simulink model "model_QK_SFSVD_ROS"  (Simulink 7.6)
settings: Solver=FixedStepDiscrete  SolverMode=SingleTasking  StartTime=0  StopTime=100  FixedStep=0.01  RelTol=1e-3
values from neighbouring files (symbols this model uses):
  parameter = block.DialogPrm(3).Data    [Kalmangain.m]    (also in init_QK_ROS.m = load('parameter'); statePrediction.m = block.DialogPrm(2).Data)
libraries: PortLib x11, simulink x2, aerolibutil x2
(part 4 of 4)

== matlab function Kalmanfilter/correction ==
  data: xpred input double; x output double; Ppred input double; y input double; sensors input double; P output double; parameter parameter double
function [x,P] = correction(xpred, Ppred, y, sensors, parameter)


R0   = parameter.R0;
Pos0 = parameter.Pos0;
B0   = parameter.B0;

x    = xpred;
P    = Ppred;
% Horizontal GPS Position
if sensors(1) == 1
    [temp, C, R] = getGPSPosition(xpred,y(1:2),R0(1:2),Pos0);
    K            = Ppred*C'*(C*Ppred*C'  +  R)^( - 1);
    x            = x  +  K*temp;
    P            = (eye(length(xpred))  -  K*C)*P;
end
% Barometric height
if sensors(2) == 1
    [temp,C,R]  =  getBarometer(xpred,y(3),R0(3));
    K           = Ppred*C'*(C*Ppred*C'  +  R)^( - 1);
    x           = x  +  K*temp;
    P           = (eye(length(xpred))  -  K*C)*P;
end
% GPS Velocity
if sensors(3) == 1
    [temp,C,R]  =  getGPSVelocity(xpred,y(4:6),R0(4:6));
    K           = Ppred*C'*(C*Ppred*C'  +  R)^( - 1);
    x           = x  +  K*temp;
    P           = (eye(length(xpred))  -  K*C)*P;
end
% Acceleration
if sensors(4) == 1
    [temp,C,R]  =  getAccelerometer(xpred,y(7:9),R0(7:9),parameter);
    K           = Ppred*C'*(C*Ppred*C'  +  R)^( - 1);
    x           = x  +  K*temp;
    P           = (eye(length(xpred))  -  K*C)*P;
end
% Gyroscope
if sensors(5) == 1
    [temp,C,R]  =  getGyroscope(xpred,y(10:12),R0(10:12));
    K           = Ppred*C'*(C*Ppred*C'  +  R)^( - 1);
    x           = x  +  K*temp;
    P           = (eye(length(xpred))  -  K*C)*P;
end
% Omega motor
if sensors(6) == 1
    [temp,C,R]  =  getOmegaMotor(xpred,y(13:16),R0(13:16));
    K           = Ppred*C'*(C*Ppred*C'  +  R)^( - 1);
    x           = x  +  K*temp;
    P           = (eye(length(xpred))  -  K*C)*P;
end
% Magnetometer
if sensors(7) == 1
    [temp, C, R] = getMagneticField(xpred,y(17:19),R0(17:19),B0);
    K            = Ppred*C'*(C*Ppred*C'  +  R)^( - 1);
    x            = x  +  K*temp;
    P            = (eye(length(xpred))  -  K*C)*P;
end
% normalize quaternions
q_0 = x(7);
q_1 = x(8);
q_2 = x(9);
q_3 = x(10);
q_length = sqrt((q_0*q_0) + (q_1*q_1) + (q_2*q_2) + (q_3*q_3));

x(7)  = x(7)/q_length;
x(8)  = x(8)/q_length;
x(9)  = x(9)/q_length;
x(10) = x(10)/q_length;

%endfunction

function [temp, C, R] = getGPSPosition(x,real_measurements,Rin,Pos0)

y = zeros(2,1);
C = zeros(2,31);
R = zeros(2);

y(1)   = Pos0(1)  +  x(1)/6378137.0/pi*180.0;                         % Latitude
y(2)   = Pos0(2)  +  x(2)/6378137.0/pi/cos(Pos0(1)*pi/180.0)*180.0;   % Longitude

C(1,1) = 180/6378137/pi;
C(2,2) = 180/6378137/pi/cos(Pos0(1)*pi/180);

R(1,1) = 180*Rin(1)/6378137/pi;
R(2,2) = 180*Rin(2)/6378137/pi/cos(Pos0(1)*pi/180);

temp   = real_measurements  -  y;

function [temp, C, R] = getGPSVelocity(x,real_measurements,Rin)

y = zeros(3,1);
C = zeros(3,31);

u = x(4);
v = x(5);
w = x(6);
q_0 = x(7);
q_1 = x(8);
q_2 = x(9);
q_3 = x(10);

y(1) = u*(q_0*q_0 + q_1*q_1 - q_2*q_2 - q_3*q_3) - v*(q_0*q_3*2.0 - q_1*q_2*2.0) + w*(q_0*q_2*2.0 + q_1*q_3*2.0);
y(2) = v*(q_0*q_0 - q_1*q_1 + q_2*q_2 - q_3*q_3) + u*(q_0*q_3*2.0 + q_1*q_2*2.0) - w*(q_0*q_1*2.0 - q_2*q_3*2.0);
y(3) = w*(q_0*q_0 - q_1*q_1 - q_2*q_2 + q_3*q_3) - u*(q_0*q_2*2.0 - q_1*q_3*2.0) + v*(q_0*q_1*2.0 + q_2*q_3*2.0);

C(1,4)  = q_0*q_0 + q_1*q_1 - q_2*q_2 - q_3*q_3;
C(1,5)  = q_0*q_3* - 2.0 + q_1*q_2*2.0;
C(1,6)  = q_0*q_2*2.0 + q_1*q_3*2.0;
C(1,7)  = q_0*u*2.0 - q_3*v*2.0 + q_2*w*2.0;
C(1,8)  = q_1*u*2.0 + q_2*v*2.0 + q_3*w*2.0;
C(1,9)  = q_2*u* - 2.0 + q_1*v*2.0 + q_0*w*2.0;
C(1,10) = q_3*u* - 2.0 - q_0*v*2.0 + q_1*w*2.0;
C(2,4)  = q_0*q_3*2.0 + q_1*q_2*2.0;
C(2,5)  = q_0*q_0 - q_1*q_1 + q_2*q_2 - q_3*q_3;
C(2,6)  = q_0*q_1* - 2.0 + q_2*q_3*2.0;
C(2,7)  = q_3*u*2.0 + q_0*v*2.0 - q_1*w*2.0;
C(2,8)  = q_2*u*2.0 - q_1*v*2.0 - q_0*w*2.0;
C(2,9)  = q_1*u*2.0 + q_2*v*2.0 + q_3*w*2.0;
C(2,10) = q_0*u*2.0 - q_3*v*2.0 + q_2*w*2.0;
C(3,4)  = q_0*q_2* - 2.0 + q_1*q_3*2.0;
C(3,5)  = q_0*q_1*2.0 + q_2*q_3*2.0;
C(3,6)  = q_0*q_0 - q_1*q_1 - q_2*q_2 + q_3*q_3;
C(3,7)  = q_2*u* - 2.0 + q_1*v*2.0 + q_0*w*2.0;
C(3,8)  = q_3*u*2.0 + q_0*v*2.0 - q_1*w*2.0;
C(3,9)  = q_0*u* - 2.0 + q_3*v*2.0 - q_2*w*2.0;
C(3,10) = q_1*u*2.0 + q_2*v*2.0 + q_3*w*2.0;

R       = diag(Rin);

temp    = real_measurements  -  y;


function [temp, C, R] = getMagneticField(x,real_measurements,Rin,B)

q_0 = x(7);
q_1 = x(8);
q_2 = x(9);
q_3 = x(10);

y       = zeros(3,1);
C       = zeros(3,31);

fieldLength             = eps  +  sqrt(B(1)*B(1) + B(2)*B(2) + B(3)*B(3));
fieldLengthMeasurement  = eps  +  sqrt(real_measurements(1)^2  +  real_measurements(2)^2  +  real_measurements(3)^2);

%% Magnetometer updates only heading angle
y(1) = (B(2)*(q_0*q_3*2.0 + q_1*q_2*2.0) - B(3)*(q_0*q_2*2.0 - q_1*q_3*2.0) + B(1)*(q_0*q_0 + q_1*q_1 - q_2*q_2 - q_3*q_3))/fieldLength;
y(2) = ( - B(1)*(q_0*q_3*2.0 - q_1*q_2*2.0) + B(3)*(q_0*q_1*2.0 + q_2*q_3*2.0) + B(2)*(q_0*q_0 - q_1*q_1 + q_2*q_2 - q_3*q_3))/fieldLength;
y(3) = (B(1)*(q_0*q_2*2.0 + q_1*q_3*2.0) - B(2)*(q_0*q_1*2.0 - q_2*q_3*2.0) + B(3)*(q_0*q_0 - q_1*q_1 - q_2*q_2 + q_3*q_3))/fieldLength;

C(1,7) =  - q_3*(q_0*(B(2)*q_0*1.0/fieldLength*2.0 - B(1)*q_3*1.0/fieldLength*2.0 + B(3)*q_1*1.0/fieldLength*2.0) + q_1*(B(1)*q_2*1.0/fieldLength*2.0 - B(2)*q_1*1.0/fieldLength*2.0 + B(3)*q_0*1.0/fieldLength*2.0) + q_2*(B(1)*q_1*1.0/fieldLength*2.0 + B(2)*q_2*1.0/fieldLength*2.0 + B(3)*q_3*1.0/fieldLength*2.0) - q_3*(B(1)*q_0*1.0/fieldLength*2.0 + B(2)*q_3*1.0/fieldLength*2.0 - B(3)*q_2*1.0/fieldLength*2.0));
C(1,8) = q_2*(q_0*(B(2)*q_0*1.0/fieldLength*2.0 - B(1)*q_3*1.0/fieldLength*2.0 + B(3)*q_1*1.0/fieldLength*2.0) + q_1*(B(1)*q_2*1.0/fieldLength*2.0 - B(2)*q_1*1.0/fieldLength*2.0 + B(3)*q_0*1.0/fieldLength*2.0) + q_2*(B(1)*q_1*1.0/fieldLength*2.0 + B(2)*q_2*1.0/fieldLength*2.0 + B(3)*q_3*1.0/fieldLength*2.0) - q_3*(B(1)*q_0*1.0/fieldLength*2.0 + B(2)*q_3*1.0/fieldLength*2.0 - B(3)*q_2*1.0/fieldLength*2.0));
C(1,9) =  - q_1*(q_0*(B(2)*q_0*1.0/fieldLength*2.0 - B(1)*q_3*1.0/fieldLength*2.0 + B(3)*q_1*1.0/fieldLength*2.0) + q_1*(B(1)*q_2*1.0/fieldLength*2.0 - B(2)*q_1*1.0/fieldLength*2.0 + B(3)*q_0*1.0/fieldLength*2.0) + q_2*(B(1)*q_1*1.0/fieldLength*2.0 + B(2)*q_2*1.0/fieldLength*2.0 + B(3)*q_3*1.0/fieldLength*2.0) - q_3*(B(1)*q_0*1.0/fieldLength*2.0 + B(2)*q_3*1.0/fieldLength*2.0 - B(3)*q_2*1.0/fieldLength*2.0));
C(1,10) = q_0*(q_0*(B(2)*q_0*1.0/fieldLength*2.0 - B(1)*q_3*1.0/fieldLength*2.0 + B(3)*q_1*1.0/fieldLength*2.0) + q_1*(B(1)*q_2*1.0/fieldLength*2.0 - B(2)*q_1*1.0/fieldLength*2.0 + B(3)*q_0*1.0/fieldLength*2.0) + q_2*(B(1)*q_1*1.0/fieldLength*2.0 + B(2)*q_2*1.0/fieldLength*2.0 + B(3)*q_3*1.0/fieldLength*2.0) - q_3*(B(1)*q_0*1.0/fieldLength*2.0 + B(2)*q_3*1.0/fieldLength*2.0 - B(3)*q_2*1.0/fieldLength*2.0));
C(2,7) = q_3*(q_0*(B(1)*q_0*1.0/fieldLength*2.0 + B(2)*q_3*1.0/fieldLength*2.0 - B(3)*q_2*1.0/fieldLength*2.0) - q_2*(B(1)*q_2*1.0/fieldLength*2.0 - B(2)*q_1*1.0/fieldLength*2.0 + B(3)*q_0*1.0/fieldLength*2.0) + q_1*(B(1)*q_1*1.0/fieldLength*2.0 + B(2)*q_2*1.0/fieldLength*2.0 + B(3)*q_3*1.0/fieldLength*2.0) + q_3*(B(2)*q_0*1.0/fieldLength*2.0 - B(1)*q_3*1.0/fieldLength*2.0 + B(3)*q_1*1.0/fieldLength*2.0));
C(2,8) =  - q_2*(q_0*(B(1)*q_0*1.0/fieldLength*2.0 + B(2)*q_3*1.0/fieldLength*2.0 - B(3)*q_2*1.0/fieldLength*2.0) - q_2*(B(1)*q_2*1.0/fieldLength*2.0 - B(2)*q_1*1.0/fieldLength*2.0 + B(3)*q_0*1.0/fieldLength*2.0) + q_1*(B(1)*q_1*1.0/fieldLength*2.0 + B(2)*q_2*1.0/fieldLength*2.0 + B(3)*q_3*1.0/fieldLength*2.0) + q_3*(B(2)*q_0*1.0/fieldLength*2.0 - B(1)*q_3*1.0/fieldLength*2.0 + B(3)*q_1*1.0/fieldLength*2.0));
C(2,9) = q_1*(q_0*(B(1)*q_0*1.0/fieldLength*2.0 + B(2)*q_3*1.0/fieldLength*2.0 - B(3)*q_2*1.0/fieldLength*2.0) - q_2*(B(1)*q_2*1.0/fieldLength*2.0 - B(2)*q_1*1.0/fieldLength*2.0 + B(3)*q_0*1.0/fieldLength*2.0) + q_1*(B(1)*q_1*1.0/fieldLength*2.0 + B(2)*q_2*1.0/fieldLength*2.0 + B(3)*q_3*1.0/fieldLength*2.0) + q_3*(B(2)*q_0*1.0/fieldLength*2.0 - B(1)*q_3*1.0/fieldLength*2.0 + B(3)*q_1*1.0/fieldLength*2.0));
C(2,10) =  - q_0*(q_0*(B(1)*q_0*1.0/fieldLength*2.0 + B(2)*q_3*1.0/fieldLength*2.0 - B(3)*q_2*1.0/fieldLength*2.0) - q_2*(B(1)*q_2*1.0/fieldLength*2.0 - B(2)*q_1*1.0/fieldLength*2.0 + B(3)*q_0*1.0/fieldLength*2.0) + q_1*(B(1)*q_1*1.0/fieldLength*2.0 + B(2)*q_2*1.0/fieldLength*2.0 + B(3)*q_3*1.0/fieldLength*2.0) + q_3*(B(2)*q_0*1.0/fieldLength*2.0 - B(1)*q_3*1.0/fieldLength*2.0 + B(3)*q_1*1.0/fieldLength*2.0));
C(3,7) = q_3*( - q_0*(B(1)*q_1*1.0/fieldLength*2.0 + B(2)*q_2*1.0/fieldLength*2.0 + B(3)*q_3*1.0/fieldLength*2.0) + q_1*(B(1)*q_0*1.0/fieldLength*2.0 + B(2)*q_3*1.0/fieldLength*2.0 - B(3)*q_2*1.0/fieldLength*2.0) + q_2*(B(2)*q_0*1.0/fieldLength*2.0 - B(1)*q_3*1.0/fieldLength*2.0 + B(3)*q_1*1.0/fieldLength*2.0) + q_3*(B(1)*q_2*1.0/fieldLength*2.0 - B(2)*q_1*1.0/fieldLength*2.0 + B(3)*q_0*1.0/fieldLength*2.0));
C(3,8) =  - q_2*( - q_0*(B(1)*q_1*1.0/fieldLength*2.0 + B(2)*q_2*1.0/fieldLength*2.0 + B(3)*q_3*1.0/fieldLength*2.0) + q_1*(B(1)*q_0*1.0/fieldLength*2.0 + B(2)*q_3*1.0/fieldLength*2.0 - B(3)*q_2*1.0/fieldLength*2.0) + q_2*(B(2)*q_0*1.0/fieldLength*2.0 - B(1)*q_3*1.0/fieldLength*2.0 + B(3)*q_1*1.0/fieldLength*2.0) + q_3*(B(1)*q_2*1.0/fieldLength*2.0 - B(2)*q_1*1.0/fieldLength*2.0 + B(3)*q_0*1.0/fieldLength*2.0));
C(3,9) = q_1*( - q_0*(B(1)*q_1*1.0/fieldLength*2.0 + B(2)*q_2*1.0/fieldLength*2.0 + B(3)*q_3*1.0/fieldLength*2.0) + q_1*(B(1)*q_0*1.0/fieldLength*2.0 + B(2)*q_3*1.0/fieldLength*2.0 - B(3)*q_2*1.0/fieldLength*2.0) + q_2*(B(2)*q_0*1.0/fieldLength*2.0 - B(1)*q_3*1.0/fieldLength*2.0 + B(3)*q_1*1.0/fieldLength*2.0) + q_3*(B(1)*q_2*1.0/fieldLength*2.0 - B(2)*q_1*1.0/fieldLength*2.0 + B(3)*q_0*1.0/fieldLength*2.0));
C(3,10) =  - q_0*( - q_0*(B(1)*q_1*1.0/fieldLength*2.0 + B(2)*q_2*1.0/fieldLength*2.0 + B(3)*q_3*1.0/fieldLength*2.0) + q_1*(B(1)*q_0*1.0/fieldLength*2.0 + B(2)*q_3*1.0/fieldLength*2.0 - B(3)*q_2*1.0/fieldLength*2.0) + q_2*(B(2)*q_0*1.0/fieldLength*2.0 - B(1)*q_3*1.0/fieldLength*2.0 + B(3)*q_1*1.0/fieldLength*2.0) + q_3*(B(1)*q_2*1.0/fieldLength*2.0 - B(2)*q_1*1.0/fieldLength*2.0 + B(3)*q_0*1.0/fieldLength*2.0));

R       = diag(Rin);

temp    = real_measurements/fieldLengthMeasurement  -  y;


function [temp,C,R] = getBarometer(x,real_measurements,Rin)

%% Initial conditions
p_z = x(3);

C      = zeros(1,31);
C(1,3) = 1.0;

R       = diag(Rin);

temp    = real_measurements  -  p_z;

function [temp,C,R] = getAccelerometer(x,real_measurements,Rin,parameter)

% parameters
g     = parameter.g;
l_m   = parameter.l_m;
m     = parameter.m;
CT2s  = parameter.CT2s;
CT1s  = parameter.CT1s;
C_wz  = parameter.C_wz;

%% Initial conditions
u = x(4);
v = x(5);
w = x(6);
q_0 = x(7);
q_1 = x(8);
q_2 = x(9);
q_3 = x(10);
a_x_bias = x(11);
a_y_bias = x(12);
a_z_bias = x(13);

p = x(17);
q = x(18);
r = x(19);
w_1 = x(20);
w_2 = x(21);
w_3 = x(22);
w_4 = x(23);

CT0s = x(25);

v_x_wind = x(29);
v_y_wind = x(30);
C_wxy    = x(31);

y     = zeros(3,1);
C     = zeros(3,31);

vx_res =  - u + v_x_wind*(q_0*q_0 + q_1*q_1 - q_2*q_2 - q_3*q_3) + v_y_wind*(q_0*q_3*2.0 + q_1*q_2*2.0);
vy_res = v - v_y_wind*(q_0*q_0 - q_1*q_1 + q_2*q_2 - q_3*q_3) + v_x_wind*(q_0*q_3*2.0 - q_1*q_2*2.0);
vz_res = w - v_x_wind*(q_0*q_2*2.0 + q_1*q_3*2.0) + v_y_wind*(q_0*q_1*2.0 - q_2*q_3*2.0);
velocityLength = eps + sqrt(vx_res^2  +  vy_res^2  +  vz_res^2);


if sum(x(20:23)) < 1500 % ground contact if motor speed is to low
    y(1) = a_x_bias + g*(q_0*q_2*2.0 - q_1*q_3*2.0);
    y(2) = a_y_bias - g*(q_0*q_1*2.0 + q_2*q_3*2.0);
    y(3) = a_z_bias - g*(q_0*q_0 - q_1*q_1 - q_2*q_2 + q_3*q_3);
    
    C(1,7) = g*q_2*2.0;
    C(1,8) = g*q_3* - 2.0;
    C(1,9) = g*q_0*2.0;
    C(1,10) = g*q_1* - 2.0;
    C(1,11) = 1.0;
    C(2,7) = g*q_1* - 2.0;
    C(2,8) = g*q_0* - 2.0;
    C(2,9) = g*q_3* - 2.0;
    C(2,10) = g*q_2* - 2.0;
    C(2,12) = 1.0;
    C(3,7) = g*q_0* - 2.0;
    C(3,8) = g*q_1*2.0;
    C(3,9) = g*q_2*2.0;
    C(3,10) = g*q_3* - 2.0;
    C(3,13) = 1.0;
else
    y(1) = a_x_bias - q*w + r*v + (C_wxy*(vx_res)*velocityLength)/m;
    y(2) = a_y_bias + p*w - r*u - (C_wxy*velocityLength*(vy_res))/m;
    y(3) = a_z_bias - p*v + q*u - (CT0s*(w_1*w_1) + CT0s*(w_2*w_2) + CT0s*(w_3*w_3) + CT0s*(w_4*w_4) - CT1s*w_2*(w + l_m*p + q_0*q_1*v_y_wind*2.0 - q_0*q_2*v_x_wind*2.0 - q_1*q_3*v_x_wind*2.0 - q_2*q_3*v_y_wind*2.0) - CT1s*w_3*(w + l_m*q + q_0*q_1*v_y_wind*2.0 - q_0*q_2*v_x_wind*2.0 - q_1*q_3*v_x_wind*2.0 - q_2*q_3*v_y_wind*2.0) + CT1s*w_4*( - w + l_m*p - q_0*q_1*v_y_wind*2.0 + q_0*q_2*v_x_wind*2.0 + q_1*q_3*v_x_wind*2.0 + q_2*q_3*v_y_wind*2.0) + CT1s*w_1*( - w + l_m*q - q_0*q_1*v_y_wind*2.0 + q_0*q_2*v_x_wind*2.0 + q_1*q_3*v_x_wind*2.0 + q_2*q_3*v_y_wind*2.0) + CT2s*abs( - w + l_m*p - q_0*q_1*v_y_wind*2.0 + q_0*q_2*v_x_wind*2.0 + q_1*q_3*v_x_wind*2.0 + q_2*q_3*v_y_wind*2.0)*( - w + l_m*p - q_0*q_1*v_y_wind*2.0 + q_0*q_2*v_x_wind*2.0 + q_1*q_3*v_x_wind*2.0 + q_2*q_3*v_y_wind*2.0) + CT2s*abs( - w + l_m*q - q_0*q_1*v_y_wind*2.0 + q_0*q_2*v_x_wind*2.0 + q_1*q_3*v_x_wind*2.0 + q_2*q_3*v_y_wind*2.0)*( - w + l_m*q - q_0*q_1*v_y_wind*2.0 + q_0*q_2*v_x_wind*2.0 + q_1*q_3*v_x_wind*2.0 + q_2*q_3*v_y_wind*2.0) - CT2s*abs(w + l_m*p + q_0*q_1*v_y_wind*2.0 - q_0*q_2*v_x_wind*2.0 - q_1*q_3*v_x_wind*2.0 - q_2*q_3*v_y_wind*2.0)*(w + l_m*p + q_0*q_1*v_y_wind*2.0 - q_0*q_2*v_x_wind*2.0 - q_1*q_3*v_x_wind*2.0 - q_2*q_3*v_y_wind*2.0) - CT2s*abs(w + l_m*q + q_0*q_1*v_y_wind*2.0 - q_0*q_2*v_x_wind*2.0 - q_1*q_3*v_x_wind*2.0 - q_2*q_3*v_y_wind*2.0)*(w + l_m*q + q_0*q_1*v_y_wind*2.0 - q_0*q_2*v_x_wind*2.0 - q_1*q_3*v_x_wind*2.0 - q_2*q_3*v_y_wind*2.0))/m - (C_wz*(vz_res)*velocityLength)/m;
    
    C(1,4) =  - (C_wxy*velocityLength)/m - (C_wxy*(vx_res)*(u* - 2.0 + v_x_wind*(q_0*q_0 + q_1*q_1 - q_2*q_2 - q_3*q_3)*2.0 + v_y_wind*(q_0*q_3*2.0 + q_1*q_2*2.0)*2.0)*1.0/velocityLength*(1.0/2.0))/m;
    C(1,5) = r + (C_wxy*(vx_res)*(v*2.0 - v_y_wind*(q_0*q_0 - q_1*q_1 + q_2*q_2 - q_3*q_3)*2.0 + v_x_wind*(q_0*q_3*2.0 - q_1*q_2*2.0)*2.0)*1.0/velocityLength*(1.0/2.0))/m;
    C(1,6) =  - q + (C_wxy*(vx_res)*(w*2.0 - v_x_wind*(q_0*q_2*2.0 + q_1*q_3*2.0)*2.0 + v_y_wind*(q_0*q_1*2.0 - q_2*q_3*2.0)*2.0)*1.0/velocityLength*(1.0/2.0))/m;
    C(1,7) = (C_wxy*(q_0*v_x_wind*2.0 + q_3*v_y_wind*2.0)*velocityLength)/m + (C_wxy*(vx_res)*((q_0*v_y_wind*2.0 - q_3*v_x_wind*2.0)*(vy_res)* - 2.0 + (q_0*v_x_wind*2.0 + q_3*v_y_wind*2.0)*(vx_res)*2.0 + (q_1*v_y_wind*2.0 - q_2*v_x_wind*2.0)*(vz_res)*2.0)*1.0/velocityLength*(1.0/2.0))/m;
    C(1,8) = (C_wxy*(q_1*v_x_wind*2.0 + q_2*v_y_wind*2.0)*velocityLength)/m + (C_wxy*(vx_res)*((q_1*v_y_wind*2.0 - q_2*v_x_wind*2.0)*(vy_res)*2.0 + (q_1*v_x_wind*2.0 + q_2*v_y_wind*2.0)*(vx_res)*2.0 + (q_0*v_y_wind*2.0 - q_3*v_x_wind*2.0)*(vz_res)*2.0)*1.0/velocityLength*(1.0/2.0))/m;
    C(1,9) = (C_wxy*(q_1*v_y_wind*2.0 - q_2*v_x_wind*2.0)*velocityLength)/m - (C_wxy*(vx_res)*((q_1*v_x_wind*2.0 + q_2*v_y_wind*2.0)*(vy_res)*2.0 - (q_1*v_y_wind*2.0 - q_2*v_x_wind*2.0)*(vx_res)*2.0 + (q_0*v_x_wind*2.0 + q_3*v_y_wind*2.0)*(vz_res)*2.0)*1.0/velocityLength*(1.0/2.0))/m;
    C(1,10) = (C_wxy*(q_0*v_y_wind*2.0 - q_3*v_x_wind*2.0)*velocityLength)/m + (C_wxy*(vx_res)*((q_0*v_x_wind*2.0 + q_3*v_y_wind*2.0)*(vy_res)*2.0 + (q_0*v_y_wind*2.0 - q_3*v_x_wind*2.0)*(vx_res)*2.0 - (q_1*v_x_wind*2.0 + q_2*v_y_wind*2.0)*(vz_res)*2.0)*1.0/velocityLength*(1.0/2.0))/m;
    C(1,11) = 1.0;
    
    %     C(1,18) =  - w;
    %     C(1,19) = v;
    %     C(1,29) = (C_wxy*velocityLength*(q_0*q_0 + q_1*q_1 - q_2*q_2 - q_3*q_3))/m + (C_wxy*(vx_res)*1.0/velocityLength*((q_0*q_3*2.0 - q_1*q_2*2.0)*(vy_res)*2.0 - (q_0*q_2*2.0 + q_1*q_3*2.0)*(vz_res)*2.0 + (vx_res)*(q_0*q_0 + q_1*q_1 - q_2*q_2 - q_3*q_3)*2.0)*(1.0/2.0))/m;
    %     C(1,30) = (C_wxy*(q_0*q_3*2.0 + q_1*q_2*2.0)*velocityLength)/m + (C_wxy*(vx_res)*1.0/velocityLength*((q_0*q_3*2.0 + q_1*q_2*2.0)*(vx_res)*2.0 - (vy_res)*(q_0*q_0 - q_1*q_1 + q_2*q_2 - q_3*q_3)*2.0 + (q_0*q_1*2.0 - q_2*q_3*2.0)*(vz_res)*2.0)*(1.0/2.0))/m;
    %     C(1,31) = ((vx_res)*velocityLength)/m;
    
    C(2,4) =  - r + (C_wxy*(u* - 2.0 + v_x_wind*(q_0*q_0 + q_1*q_1 - q_2*q_2 - q_3*q_3)*2.0 + v_y_wind*(q_0*q_3*2.0 + q_1*q_2*2.0)*2.0)*1.0/velocityLength*(vy_res)*(1.0/2.0))/m;
    C(2,5) =  - (C_wxy*velocityLength)/m - (C_wxy*(v*2.0 - v_y_wind*(q_0*q_0 - q_1*q_1 + q_2*q_2 - q_3*q_3)*2.0 + v_x_wind*(q_0*q_3*2.0 - q_1*q_2*2.0)*2.0)*1.0/velocityLength*(vy_res)*(1.0/2.0))/m;
    C(2,6) = p - (C_wxy*(w*2.0 - v_x_wind*(q_0*q_2*2.0 + q_1*q_3*2.0)*2.0 + v_y_wind*(q_0*q_1*2.0 - q_2*q_3*2.0)*2.0)*1.0/velocityLength*(vy_res)*(1.0/2.0))/m;
    C(2,7) = (C_wxy*(q_0*v_y_wind*2.0 - q_3*v_x_wind*2.0)*velocityLength)/m - (C_wxy*((q_0*v_y_wind*2.0 - q_3*v_x_wind*2.0)*(vy_res)* - 2.0 + (q_0*v_x_wind*2.0 + q_3*v_y_wind*2.0)*(vx_res)*2.0 + (q_1*v_y_wind*2.0 - q_2*v_x_wind*2.0)*(vz_res)*2.0)*1.0/velocityLength*(vy_res)*(1.0/2.0))/m;
    C(2,8) =  - (C_wxy*(q_1*v_y_wind*2.0 - q_2*v_x_wind*2.0)*velocityLength)/m - (C_wxy*((q_1*v_y_wind*2.0 - q_2*v_x_wind*2.0)*(vy_res)*2.0 + (q_1*v_x_wind*2.0 + q_2*v_y_wind*2.0)*(vx_res)*2.0 + (q_0*v_y_wind*2.0 - q_3*v_x_wind*2.0)*(vz_res)*2.0)*1.0/velocityLength*(vy_res)*(1.0/2.0))/m;
    C(2,9) = (C_wxy*(q_1*v_x_wind*2.0 + q_2*v_y_wind*2.0)*velocityLength)/m + (C_wxy*((q_1*v_x_wind*2.0 + q_2*v_y_wind*2.0)*(vy_res)*2.0 - (q_1*v_y_wind*2.0 - q_2*v_x_wind*2.0)*(vx_res)*2.0 + (q_0*v_x_wind*2.0 + q_3*v_y_wind*2.0)*(vz_res)*2.0)*1.0/velocityLength*(vy_res)*(1.0/2.0))/m;
    C(2,10) =  - (C_wxy*(q_0*v_x_wind*2.0 + q_3*v_y_wind*2.0)*velocityLength)/m - (C_wxy*((q_0*v_x_wind*2.0 + q_3*v_y_wind*2.0)*(vy_res)*2.0 + (q_0*v_y_wind*2.0 - q_3*v_x_wind*2.0)*(vx_res)*2.0 - (q_1*v_x_wind*2.0 + q_2*v_y_wind*2.0)*(vz_res)*2.0)*1.0/velocityLength*(vy_res)*(1.0/2.0))/m;
    C(2,12) = 1.0;
    
    %     C(2,17) = w;
    %     C(2,19) =  - u;
    %     C(2,29) =  - (C_wxy*(q_0*q_3*2.0 - q_1*q_2*2.0)*velocityLength)/m - (C_wxy*1.0/velocityLength*(vy_res)*((q_0*q_3*2.0 - q_1*q_2*2.0)*(vy_res)*2.0 - (q_0*q_2*2.0 + q_1*q_3*2.0)*(vz_res)*2.0 + (vx_res)*(q_0*q_0 + q_1*q_1 - q_2*q_2 - q_3*q_3)*2.0)*(1.0/2.0))/m;
    %     C(2,30) = (C_wxy*velocityLength*(q_0*q_0 - q_1*q_1 + q_2*q_2 - q_3*q_3))/m - (C_wxy*1.0/velocityLength*(vy_res)*((q_0*q_3*2.0 + q_1*q_2*2.0)*(vx_res)*2.0 - (vy_res)*(q_0*q_0 - q_1*q_1 + q_2*q_2 - q_3*q_3)*2.0 + (q_0*q_1*2.0 - q_2*q_3*2.0)*(vz_res)*2.0)*(1.0/2.0))/m;
    %     C(2,31) =  - (velocityLength*(vy_res))/m;
    
    C(3,4) = q + (C_wz*(u* - 2.0 + v_x_wind*(q_0*q_0 + q_1*q_1 - q_2*q_2 - q_3*q_3)*2.0 + v_y_wind*(q_0*q_3*2.0 + q_1*q_2*2.0)*2.0)*(vz_res)*1.0/velocityLength*(1.0/2.0))/m;
    C(3,5) =  - p - (C_wz*(v*2.0 - v_y_wind*(q_0*q_0 - q_1*q_1 + q_2*q_2 - q_3*q_3)*2.0 + v_x_wind*(q_0*q_3*2.0 - q_1*q_2*2.0)*2.0)*(vz_res)*1.0/velocityLength*(1.0/2.0))/m;
    C(3,6) = (CT1s*w_1 + CT1s*w_2 + CT1s*w_3 + CT1s*w_4 + CT2s*abs( - w + l_m*p - q_0*q_1*v_y_wind*2.0 + q_0*q_2*v_x_wind*2.0 + q_1*q_3*v_x_wind*2.0 + q_2*q_3*v_y_wind*2.0) + CT2s*abs( - w + l_m*q - q_0*q_1*v_y_wind*2.0 + q_0*q_2*v_x_wind*2.0 + q_1*q_3*v_x_wind*2.0 + q_2*q_3*v_y_wind*2.0) + CT2s*abs(w + l_m*p + q_0*q_1*v_y_wind*2.0 - q_0*q_2*v_x_wind*2.0 - q_1*q_3*v_x_wind*2.0 - q_2*q_3*v_y_wind*2.0) + CT2s*abs(w + l_m*q + q_0*q_1*v_y_wind*2.0 - q_0*q_2*v_x_wind*2.0 - q_1*q_3*v_x_wind*2.0 - q_2*q_3*v_y_wind*2.0) + CT2s*(((w + l_m*q + q_0*q_1*v_y_wind*2.0 - q_0*q_2*v_x_wind*2.0 - q_1*q_3*v_x_wind*2.0 - q_2*q_3*v_y_wind*2.0)/abs(w + l_m*q + q_0*q_1*v_y_wind*2.0 - q_0*q_2*v_x_wind*2.0 - q_1*q_3*v_x_wind*2.0 - q_2*q_3*v_y_wind*2.0)))*(w + l_m*q + q_0*q_1*v_y_wind*2.0 - q_0*q_2*v_x_wind*2.0 - q_1*q_3*v_x_wind*2.0 - q_2*q_3*v_y_wind*2.0) + CT2s*((( - w + l_m*p - q_0*q_1*v_y_wind*2.0 + q_0*q_2*v_x_wind*2.0 + q_1*q_3*v_x_wind*2.0 + q_2*q_3*v_y_wind*2.0)/abs( - w + l_m*p - q_0*q_1*v_y_wind*2.0 + q_0*q_2*v_x_wind*2.0 + q_1*q_3*v_x_wind*2.0 + q_2*q_3*v_y_wind*2.0)))*( - w + l_m*p - q_0*q_1*v_y_wind*2.0 + q_0*q_2*v_x_wind*2.0 + q_1*q_3*v_x_wind*2.0 + q_2*q_3*v_y_wind*2.0) + CT2s*((( - w + l_m*q - q_0*q_1*v_y_wind*2.0 + q_0*q_2*v_x_wind*2.0 + q_1*q_3*v_x_wind*2.0 + q_2*q_3*v_y_wind*2.0)/abs( - w + l_m*q - q_0*q_1*v_y_wind*2.0 + q_0*q_2*v_x_wind*2.0 + q_1*q_3*v_x_wind*2.0 + q_2*q_3*v_y_wind*2.0)))*( - w + l_m*q - q_0*q_1*v_y_wind*2.0 + q_0*q_2*v_x_wind*2.0 + q_1*q_3*v_x_wind*2.0 + q_2*q_3*v_y_wind*2.0) + CT2s*(((w + l_m*p + q_0*q_1*v_y_wind*2.0 - q_0*q_2*v_x_wind*2.0 - q_1*q_3*v_x_wind*2.0 - q_2*q_3*v_y_wind*2.0)/abs(w + l_m*p + q_0*q_1*v_y_wind*2.0 - q_0*q_2*v_x_wind*2.0 - q_1*q_3*v_x_wind*2.0 - q_2*q_3*v_y_wind*2.0)))*(w + l_m*p + q_0*q_1*v_y_wind*2.0 - q_0*q_2*v_x_wind*2.0 - q_1*q_3*v_x_wind*2.0 - q_2*q_3*v_y_wind*2.0))/m - (C_wz*velocityLength)/m - (C_wz*(vz_res)*(w*2.0 - v_x_wind*(q_0*q_2*2.0 + q_1*q_3*2.0)*2.0 + v_y_wind*(q_0*q_1*2.0 - q_2*q_3*2.0)*2.0)*1.0/velocityLength*(1.0/2.0))/m;
    C(3,7) = (CT1s*w_1*(q_1*v_y_wind*2.0 - q_2*v_x_wind*2.0) + CT1s*w_2*(q_1*v_y_wind*2.0 - q_2*v_x_wind*2.0) + CT1s*w_3*(q_1*v_y_wind*2.0 - q_2*v_x_wind*2.0) + CT1s*w_4*(q_1*v_y_wind*2.0 - q_2*v_x_wind*2.0) + CT2s*abs( - w + l_m*p - q_0*q_1*v_y_wind*2.0 + q_0*q_2*v_x_wind*2.0 + q_1*q_3*v_x_wind*2.0 + q_2*q_3*v_y_wind*2.0)*(q_1*v_y_wind*2.0 - q_2*v_x_wind*2.0) + CT2s*abs( - w + l_m*q - q_0*q_1*v_y_wind*2.0 + q_0*q_2*v_x_wind*2.0 + q_1*q_3*v_x_wind*2.0 + q_2*q_3*v_y_wind*2.0)*(q_1*v_y_wind*2.0 - q_2*v_x_wind*2.0) + CT2s*abs(w + l_m*p + q_0*q_1*v_y_wind*2.0 - q_0*q_2*v_x_wind*2.0 - q_1*q_3*v_x_wind*2.0 - q_2*q_3*v_y_wind*2.0)*(q_1*v_y_wind*2.0 - q_2*v_x_wind*2.0) + CT2s*abs(w + l_m*q + q_0*q_1*v_y_wind*2.0 - q_0*q_2*v_x_wind*2.0 - q_1*q_3*v_x_wind*2.0 - q_2*q_3*v_y_wind*2.0)*(q_1*v_y_wind*2.0 - q_2*v_x_wind*2.0) + CT2s*((( - w + l_m*p - q_0*q_1*v_y_wind*2.0 + q_0*q_2*v_x_wind*2.0 + q_1*q_3*v_x_wind*2.0 + q_2*q_3*v_y_wind*2.0)/abs( - w + l_m*p - q_0*q_1*v_y_wind*2.0 + q_0*q_2*v_x_wind*2.0 + q_1*q_3*v_x_wind*2.0 + q_2*q_3*v_y_wind*2.0)))*(q_1*v_y_wind*2.0 - q_2*v_x_wind*2.0)*( - w + l_m*p - q_0*q_1*v_y_wind*2.0 + q_0*q_2*v_x_wind*2.0 + q_1*q_3*v_x_wind*2.0 + q_2*q_3*v_y_wind*2.0) + CT2s*((( - w + l_m*q - q_0*q_1*v_y_wind*2.0 + q_0*q_2*v_x_wind*2.0 + q_1*q_3*v_x_wind*2.0 + q_2*q_3*v_y_wind*2.0)/abs( - w + l_m*q - q_0*q_1*v_y_wind*2.0 + q_0*q_2*v_x_wind*2.0 + q_1*q_3*v_x_wind*2.0 + q_2*q_3*v_y_wind*2.0)))*(q_1*v_y_wind*2.0 - q_2*v_x_wind*2.0)*( - w + l_m*q - q_0*q_1*v_y_wind*2.0 + q_0*q_2*v_x_wind*2.0 + q_1*q_3*v_x_wind*2.0 + q_2*q_3*v_y_wind*2.0) + CT2s*(((w + l_m*p + q_0*q_1*v_y_wind*2.0 - q_0*q_2*v_x_wind*2.0 - q_1*q_3*v_x_wind*2.0 - q_2*q_3*v_y_wind*2.0)/abs(w + l_m*p + q_0*q_1*v_y_wind*2.0 - q_0*q_2*v_x_wind*2.0 - q_1*q_3*v_x_wind*2.0 - q_2*q_3*v_y_wind*2.0)))*(q_1*v_y_wind*2.0 - q_2*v_x_wind*2.0)*(w + l_m*p + q_0*q_1*v_y_wind*2.0 - q_0*q_2*v_x_wind*2.0 - q_1*q_3*v_x_wind*2.0 - q_2*q_3*v_y_wind*2.0) + CT2s*(((w + l_m*q + q_0*q_1*v_y_wind*2.0 - q_0*q_2*v_x_wind*2.0 - q_1*q_3*v_x_wind*2.0 - q_2*q_3*v_y_wind*2.0)/abs(w + l_m*q + q_0*q_1*v_y_wind*2.0 - q_0*q_2*v_x_wind*2.0 - q_1*q_3*v_x_wind*2.0 - q_2*q_3*v_y_wind*2.0)))*(q_1*v_y_wind*2.0 - q_2*v_x_wind*2.0)*(w + l_m*q + q_0*q_1*v_y_wind*2.0 - q_0*q_2*v_x_wind*2.0 - q_1*q_3*v_x_wind*2.0 - q_2*q_3*v_y_wind*2.0))/m - (C_wz*(q_1*v_y_wind*2.0 - q_2*v_x_wind*2.0)*velocityLength)/m - (C_wz*(vz_res)*((q_0*v_y_wind*2.0 - q_3*v_x_wind*2.0)*(vy_res)* - 2.0 + (q_0*v_x_wind*2.0 + q_3*v_y_wind*2.0)*(vx_res)*2.0 + (q_1*v_y_wind*2.0 - q_2*v_x_wind*2.0)*(vz_res)*2.0)*1.0/velocityLength*(1.0/2.0))/m;
    C(3,8) = (CT1s*w_1*(q_0*v_y_wind*2.0 - q_3*v_x_wind*2.0) + CT1s*w_2*(q_0*v_y_wind*2.0 - q_3*v_x_wind*2.0) + CT1s*w_3*(q_0*v_y_wind*2.0 - q_3*v_x_wind*2.0) + CT1s*w_4*(q_0*v_y_wind*2.0 - q_3*v_x_wind*2.0) + CT2s*abs( - w + l_m*p - q_0*q_1*v_y_wind*2.0 + q_0*q_2*v_x_wind*2.0 + q_1*q_3*v_x_wind*2.0 + q_2*q_3*v_y_wind*2.0)*(q_0*v_y_wind*2.0 - q_3*v_x_wind*2.0) + CT2s*abs( - w + l_m*q - q_0*q_1*v_y_wind*2.0 + q_0*q_2*v_x_wind*2.0 + q_1*q_3*v_x_wind*2.0 + q_2*q_3*v_y_wind*2.0)*(q_0*v_y_wind*2.0 - q_3*v_x_wind*2.0) + CT2s*abs(w + l_m*p + q_0*q_1*v_y_wind*2.0 - q_0*q_2*v_x_wind*2.0 - q_1*q_3*v_x_wind*2.0 - q_2*q_3*v_y_wind*2.0)*(q_0*v_y_wind*2.0 - q_3*v_x_wind*2.0) + CT2s*abs(w + l_m*q + q_0*q_1*v_y_wind*2.0 - q_0*q_2*v_x_wind*2.0 - q_1*q_3*v_x_wind*2.0 - q_2*q_3*v_y_wind*2.0)*(q_0*v_y_wind*2.0 - q_3*v_x_wind*2.0) + CT2s*((( - w + l_m*p - q_0*q_1*v_y_wind*2.0 + q_0*q_2*v_x_wind*2.0 + q_1*q_3*v_x_wind*2.0 + q_2*q_3*v_y_wind*2.0)/abs( - w + l_m*p - q_0*q_1*v_y_wind*2.0 + q_0*q_2*v_x_wind*2.0 + q_1*q_3*v_x_wind*2.0 + q_2*q_3*v_y_wind*2.0)))*(q_0*v_y_wind*2.0 - q_3*v_x_wind*2.0)*( - w + l_m*p - q_0*q_1*v_y_wind*2.0 + q_0*q_2*v_x_wind*2.0 + q_1*q_3*v_x_wind*2.0 + q_2*q_3*v_y_wind*2.0) + CT2s*((( - w + l_m*q - q_0*q_1*v_y_wind*2.0 + q_0*q_2*v_x_wind*2.0 + q_1*q_3*v_x_wind*2.0 + q_2*q_3*v_y_wind*2.0)/abs( - w + l_m*q - q_0*q_1*v_y_wind*2.0 + q_0*q_2*v_x_wind*2.0 + q_1*q_3*v_x_wind*2.0 + q_2*q_3*v_y_wind*2.0)))*(q_0*v_y_wind*2.0 - q_3*v_x_wind*2.0)*( - w + l_m*q - q_0*q_1*v_y_wind*2.0 + q_0*q_2*v_x_wind*2.0 + q_1*q_3*v_x_wind*2.0 + q_2*q_3*v_y_wind*2.0) + CT2s*(((w + l_m*p + q_0*q_1*v_y_wind*2.0 - q_0*q_2*v_x_wind*2.0 - q_1*q_3*v_x_wind*2.0 - q_2*q_3*v_y_wind*2.0)/abs(w + l_m*p + q_0*q_1*v_y_wind*2.0 - q_0*q_2*v_x_wind*2.0 - q_1*q_3*v_x_wind*2.0 - q_2*q_3*v_y_wind*2.0)))*(q_0*v_y_wind*2.0 - q_3*v_x_wind*2.0)*(w + l_m*p + q_0*q_1*v_y_wind*2.0 - q_0*q_2*v_x_wind*2.0 - q_1*q_3*v_x_wind*2.0 - q_2*q_3*v_y_wind*2.0) + CT2s*(((w + l_m*q + q_0*q_1*v_y_wind*2.0 - q_0*q_2*v_x_wind*2.0 - q_1*q_3*v_x_wind*2.0 - q_2*q_3*v_y_wind*2.0)/abs(w + l_m*q + q_0*q_1*v_y_wind*2.0 - q_0*q_2*v_x_wind*2.0 - q_1*q_3*v_x_wind*2.0 - q_2*q_3*v_y_wind*2.0)))*(q_0*v_y_wind*2.0 - q_3*v_x_wind*2.0)*(w + l_m*q + q_0*q_1*v_y_wind*2.0 - q_0*q_2*v_x_wind*2.0 - q_1*q_3*v_x_wind*2.0 - q_2*q_3*v_y_wind*2.0))/m - (C_wz*(q_0*v_y_wind*2.0 - q_3*v_x_wind*2.0)*velocityLength)/m - (C_wz*(vz_res)*((q_1*v_y_wind*2.0 - q_2*v_x_wind*2.0)*(vy_res)*2.0 + (q_1*v_x_wind*2.0 + q_2*v_y_wind*2.0)*(vx_res)*2.0 + (q_0*v_y_wind*2.0 - q_3*v_x_wind*2.0)*(vz_res)*2.0)*1.0/velocityLength*(1.0/2.0))/m;
    C(3,9) =  - (CT1s*w_1*(q_0*v_x_wind*2.0 + q_3*v_y_wind*2.0) + CT1s*w_2*(q_0*v_x_wind*2.0 + q_3*v_y_wind*2.0) + CT1s*w_3*(q_0*v_x_wind*2.0 + q_3*v_y_wind*2.0) + CT1s*w_4*(q_0*v_x_wind*2.0 + q_3*v_y_wind*2.0) + CT2s*abs( - w + l_m*p - q_0*q_1*v_y_wind*2.0 + q_0*q_2*v_x_wind*2.0 + q_1*q_3*v_x_wind*2.0 + q_2*q_3*v_y_wind*2.0)*(q_0*v_x_wind*2.0 + q_3*v_y_wind*2.0) + CT2s*abs( - w + l_m*q - q_0*q_1*v_y_wind*2.0 + q_0*q_2*v_x_wind*2.0 + q_1*q_3*v_x_wind*2.0 + q_2*q_3*v_y_wind*2.0)*(q_0*v_x_wind*2.0 + q_3*v_y_wind*2.0) + CT2s*abs(w + l_m*p + q_0*q_1*v_y_wind*2.0 - q_0*q_2*v_x_wind*2.0 - q_1*q_3*v_x_wind*2.0 - q_2*q_3*v_y_wind*2.0)*(q_0*v_x_wind*2.0 + q_3*v_y_wind*2.0) + CT2s*abs(w + l_m*q + q_0*q_1*v_y_wind*2.0 - q_0*q_2*v_x_wind*2.0 - q_1*q_3*v_x_wind*2.0 - q_2*q_3*v_y_wind*2.0)*(q_0*v_x_wind*2.0 + q_3*v_y_wind*2.0) + CT2s*((( - w + l_m*p - q_0*q_1*v_y_wind*2.0 + q_0*q_2*v_x_wind*2.0 + q_1*q_3*v_x_wind*2.0 + q_2*q_3*v_y_wind*2.0)/abs( - w + l_m*p - q_0*q_1*v_y_wind*2.0 + q_0*q_2*v_x_wind*2.0 + q_1*q_3*v_x_wind*2.0 + q_2*q_3*v_y_wind*2.0)))*(q_0*v_x_wind*2.0 + q_3*v_y_wind*2.0)*( - w + l_m*p - q_0*q_1*v_y_wind*2.0 + q_0*q_2*v_x_wind*2.0 + q_1*q_3*v_x_wind*2.0 + q_2*q_3*v_y_wind*2.0) + CT2s*((( - w + l_m*q - q_0*q_1*v_y_wind*2.0 + q_0*q_2*v_x_wind*2.0 + q_1*q_3*v_x_wind*2.0 + q_2*q_3*v_y_wind*2.0)/abs( - w + l_m*q - q_0*q_1*v_y_wind*2.0 + q_0*q_2*v_x_wind*2.0 + q_1*q_3*v_x_wind*2.0 + q_2*q_3*v_y_wind*2.0)))*(q_0*v_x_wind*2.0 + q_3*v_y_wind*2.0)*( - w + l_m*q - q_0*q_1*v_y_wind*2.0 + q_0*q_2*v_x_wind*2.0 + q_1*q_3*v_x_wind*2.0 + q_2*q_3*v_y_wind*2.0) + CT2s*(((w + l_m*p + q_0*q_1*v_y_wind*2.0 - q_0*q_2*v_x_wind*2.0 - q_1*q_3*v_x_wind*2.0 - q_2*q_3*v_y_wind*2.0)/abs(w + l_m*p + q_0*q_1*v_y_wind*2.0 - q_0*q_2*v_x_wind*2.0 - q_1*q_3*v_x_wind*2.0 - q_2*q_3*v_y_wind*2.0)))*(q_0*v_x_wind*2.0 + q_3*v_y_wind*2.0)*(w + l_m*p + q_0*q_1*v_y_wind*2.0 - q_0*q_2*v_x_wind*2.0 - q_1*q_3*v_x_wind*2.0 - q_2*q_3*v_y_wind*2.0) + CT2s*(((w + l_m*q + q_0*q_1*v_y_wind*2.0 - q_0*q_2*v_x_wind*2.0 - q_1*q_3*v_x_wind*2.0 - q_2*q_3*v_y_wind*2.0)/abs(w + l_m*q + q_0*q_1*v_y_wind*2.0 - q_0*q_2*v_x_wind*2.0 - q_1*q_3*v_x_wind*2.0 - q_2*q_3*v_y_wind*2.0)))*(q_0*v_x_wind*2.0 + q_3*v_y_wind*2.0)*(w + l_m*q + q_0*q_1*v_y_wind*2.0 - q_0*q_2*v_x_wind*2.0 - q_1*q_3*v_x_wind*2.0 - q_2*q_3*v_y_wind*2.0))/m + (C_wz*(q_0*v_x_wind*2.0 + q_3*v_y_wind*2.0)*velocityLength)/m + (C_wz*(vz_res)*((q_1*v_x_wind*2.0 + q_2*v_y_wind*2.0)*(vy_res)*2.0 - (q_1*v_y_wind*2.0 - q_2*v_x_wind*2.0)*(vx_res)*2.0 + (q_0*v_x_wind*2.0 + q_3*v_y_wind*2.0)*(vz_res)*2.0)*1.0/velocityLength*(1.0/2.0))/m;
    C(3,10) =  - (CT1s*w_1*(q_1*v_x_wind*2.0 + q_2*v_y_wind*2.0) + CT1s*w_2*(q_1*v_x_wind*2.0 + q_2*v_y_wind*2.0) + CT1s*w_3*(q_1*v_x_wind*2.0 + q_2*v_y_wind*2.0) + CT1s*w_4*(q_1*v_x_wind*2.0 + q_2*v_y_wind*2.0) + CT2s*abs( - w + l_m*p - q_0*q_1*v_y_wind*2.0 + q_0*q_2*v_x_wind*2.0 + q_1*q_3*v_x_wind*2.0 + q_2*q_3*v_y_wind*2.0)*(q_1*v_x_wind*2.0 + q_2*v_y_wind*2.0) + CT2s*abs( - w + l_m*q - q_0*q_1*v_y_wind*2.0 + q_0*q_2*v_x_wind*2.0 + q_1*q_3*v_x_wind*2.0 + q_2*q_3*v_y_wind*2.0)*(q_1*v_x_wind*2.0 + q_2*v_y_wind*2.0) + CT2s*abs(w + l_m*p + q_0*q_1*v_y_wind*2.0 - q_0*q_2*v_x_wind*2.0 - q_1*q_3*v_x_wind*2.0 - q_2*q_3*v_y_wind*2.0)*(q_1*v_x_wind*2.0 + q_2*v_y_wind*2.0) + CT2s*abs(w + l_m*q + q_0*q_1*v_y_wind*2.0 - q_0*q_2*v_x_wind*2.0 - q_1*q_3*v_x_wind*2.0 - q_2*q_3*v_y_wind*2.0)*(q_1*v_x_wind*2.0 + q_2*v_y_wind*2.0) + CT2s*((( - w + l_m*p - q_0*q_1*v_y_wind*2.0 + q_0*q_2*v_x_wind*2.0 + q_1*q_3*v_x_wind*2.0 + q_2*q_3*v_y_wind*2.0)/abs( - w + l_m*p - q_0*q_1*v_y_wind*2.0 + q_0*q_2*v_x_wind*2.0 + q_1*q_3*v_x_wind*2.0 + q_2*q_3*v_y_wind*2.0)))*(q_1*v_x_wind*2.0 + q_2*v_y_wind*2.0)*( - w + l_m*p - q_0*q_1*v_y_wind*2.0 + q_0*q_2*v_x_wind*2.0 + q_1*q_3*v_x_wind*2.0 + q_2*q_3*v_y_wind*2.0) + CT2s*((( - w + l_m*q - q_0*q_1*v_y_wind*2.0 + q_0*q_2*v_x_wind*2.0 + q_1*q_3*v_x_wind*2.0 + q_2*q_3*v_y_wind*2.0)/abs( - w + l_m*q - q_0*q_1*v_y_wind*2.0 + q_0*q_2*v_x_wind*2.0 + q_1*q_3*v_x_wind*2.0 + q_2*q_3*v_y_wind*2.0)))*(q_1*v_x_wind*2.0 + q_2*v_y_wind*2.0)*( - w + l_m*q - q_0*q_1*v_y_wind*2.0 + q_0*q_2*v_x_wind*2.0 + q_1*q_3*v_x_wind*2.0 + q_2*q_3*v_y_wind*2.0) + CT2s*(((w + l_m*p + q_0*q_1*v_y_wind*2.0 - q_0*q_2*v_x_wind*2.0 - q_1*q_3*v_x_wind*2.0 - q_2*q_3*v_y_wind*2.0)/abs(w + l_m*p + q_0*q_1*v_y_wind*2.0 - q_0*q_2*v_x_wind*2.0 - q_1*q_3*v_x_wind*2.0 - q_2*q_3*v_y_wind*2.0)))*(q_1*v_x_wind*2.0 + q_2*v_y_wind*2.0)*(w + l_m*p + q_0*q_1*v_y_wind*2.0 - q_0*q_2*v_x_wind*2.0 - q_1*q_3*v_x_wind*2.0 - q_2*q_3*v_y_wind*2.0) + CT2s*(((w + l_m*q + q_0*q_1*v_y_wind*2.0 - q_0*q_2*v_x_wind*2.0 - q_1*q_3*v_x_wind*2.0 - q_2*q_3*v_y_wind*2.0)/abs(w + l_m*q + q_0*q_1*v_y_wind*2.0 - q_0*q_2*v_x_wind*2.0 - q_1*q_3*v_x_wind*2.0 - q_2*q_3*v_y_wind*2.0)))*(q_1*v_x_wind*2.0 + q_2*v_y_wind*2.0)*(w + l_m*q + q_0*q_1*v_y_wind*2.0 - q_0*q_2*v_x_wind*2.0 - q_1*q_3*v_x_wind*2.0 - q_2*q_3*v_y_wind*2.0))/m + (C_wz*(q_1*v_x_wind*2.0 + q_2*v_y_wind*2.0)*velocityLength)/m - (C_wz*(vz_res)*((q_0*v_x_wind*2.0 + q_3*v_y_wind*2.0)*(vy_res)*2.0 + (q_0*v_y_wind*2.0 - q_3*v_x_wind*2.0)*(vx_res)*2.0 - (q_1*v_x_wind*2.0 + q_2*v_y_wind*2.0)*(vz_res)*2.0)*1.0/velocityLength*(1.0/2.0))/m;
    C(3,13) = 1.0;
    
    %     C(3,17) =  - v + (CT2s*l_m*abs(w + l_m*p + q_0*q_1*v_y_wind*2.0 - q_0*q_2*v_x_wind*2.0 - q_1*q_3*v_x_wind*2.0 - q_2*q_3*v_y_wind*2.0) + CT1s*l_m*w_2 - CT1s*l_m*w_4 - CT2s*l_m*abs( - w + l_m*p - q_0*q_1*v_y_wind*2.0 + q_0*q_2*v_x_wind*2.0 + q_1*q_3*v_x_wind*2.0 + q_2*q_3*v_y_wind*2.0) - CT2s*l_m*((( - w + l_m*p - q_0*q_1*v_y_wind*2.0 + q_0*q_2*v_x_wind*2.0 + q_1*q_3*v_x_wind*2.0 + q_2*q_3*v_y_wind*2.0)/abs( - w + l_m*p - q_0*q_1*v_y_wind*2.0 + q_0*q_2*v_x_wind*2.0 + q_1*q_3*v_x_wind*2.0 + q_2*q_3*v_y_wind*2.0)))*( - w + l_m*p - q_0*q_1*v_y_wind*2.0 + q_0*q_2*v_x_wind*2.0 + q_1*q_3*v_x_wind*2.0 + q_2*q_3*v_y_wind*2.0) + CT2s*l_m*(((w + l_m*p + q_0*q_1*v_y_wind*2.0 - q_0*q_2*v_x_wind*2.0 - q_1*q_3*v_x_wind*2.0 - q_2*q_3*v_y_wind*2.0)/abs(w + l_m*p + q_0*q_1*v_y_wind*2.0 - q_0*q_2*v_x_wind*2.0 - q_1*q_3*v_x_wind*2.0 - q_2*q_3*v_y_wind*2.0)))*(w + l_m*p + q_0*q_1*v_y_wind*2.0 - q_0*q_2*v_x_wind*2.0 - q_1*q_3*v_x_wind*2.0 - q_2*q_3*v_y_wind*2.0))/m;
    %     C(3,18) = u + (CT2s*l_m*abs(w + l_m*q + q_0*q_1*v_y_wind*2.0 - q_0*q_2*v_x_wind*2.0 - q_1*q_3*v_x_wind*2.0 - q_2*q_3*v_y_wind*2.0) - CT1s*l_m*w_1 + CT1s*l_m*w_3 - CT2s*l_m*abs( - w + l_m*q - q_0*q_1*v_y_wind*2.0 + q_0*q_2*v_x_wind*2.0 + q_1*q_3*v_x_wind*2.0 + q_2*q_3*v_y_wind*2.0) - CT2s*l_m*((( - w + l_m*q - q_0*q_1*v_y_wind*2.0 + q_0*q_2*v_x_wind*2.0 + q_1*q_3*v_x_wind*2.0 + q_2*q_3*v_y_wind*2.0)/abs( - w + l_m*q - q_0*q_1*v_y_wind*2.0 + q_0*q_2*v_x_wind*2.0 + q_1*q_3*v_x_wind*2.0 + q_2*q_3*v_y_wind*2.0)))*( - w + l_m*q - q_0*q_1*v_y_wind*2.0 + q_0*q_2*v_x_wind*2.0 + q_1*q_3*v_x_wind*2.0 + q_2*q_3*v_y_wind*2.0) + CT2s*l_m*(((w + l_m*q + q_0*q_1*v_y_wind*2.0 - q_0*q_2*v_x_wind*2.0 - q_1*q_3*v_x_wind*2.0 - q_2*q_3*v_y_wind*2.0)/abs(w + l_m*q + q_0*q_1*v_y_wind*2.0 - q_0*q_2*v_x_wind*2.0 - q_1*q_3*v_x_wind*2.0 - q_2*q_3*v_y_wind*2.0)))*(w + l_m*q + q_0*q_1*v_y_wind*2.0 - q_0*q_2*v_x_wind*2.0 - q_1*q_3*v_x_wind*2.0 - q_2*q_3*v_y_wind*2.0))/m;
    %     C(3,20) =  - (CT0s*w_1*2.0 + CT1s*( - w + l_m*q - q_0*q_1*v_y_wind*2.0 + q_0*q_2*v_x_wind*2.0 + q_1*q_3*v_x_wind*2.0 + q_2*q_3*v_y_wind*2.0))/m;
    %     C(3,21) =  - (CT0s*w_2*2.0 - CT1s*(w + l_m*p + q_0*q_1*v_y_wind*2.0 - q_0*q_2*v_x_wind*2.0 - q_1*q_3*v_x_wind*2.0 - q_2*q_3*v_y_wind*2.0))/m;
    %     C(3,22) =  - (CT0s*w_3*2.0 - CT1s*(w + l_m*q + q_0*q_1*v_y_wind*2.0 - q_0*q_2*v_x_wind*2.0 - q_1*q_3*v_x_wind*2.0 - q_2*q_3*v_y_wind*2.0))/m;
    %     C(3,23) =  - (CT0s*w_4*2.0 + CT1s*( - w + l_m*p - q_0*q_1*v_y_wind*2.0 + q_0*q_2*v_x_wind*2.0 + q_1*q_3*v_x_wind*2.0 + q_2*q_3*v_y_wind*2.0))/m;
    %     C(3,25) =  - (w_1*w_1 + w_2*w_2 + w_3*w_3 + w_4*w_4)/m;
    %     C(3,29) =  - (CT2s*abs( - w + l_m*p - q_0*q_1*v_y_wind*2.0 + q_0*q_2*v_x_wind*2.0 + q_1*q_3*v_x_wind*2.0 + q_2*q_3*v_y_wind*2.0)*(q_0*q_2*2.0 + q_1*q_3*2.0) + CT2s*abs( - w + l_m*q - q_0*q_1*v_y_wind*2.0 + q_0*q_2*v_x_wind*2.0 + q_1*q_3*v_x_wind*2.0 + q_2*q_3*v_y_wind*2.0)*(q_0*q_2*2.0 + q_1*q_3*2.0) + CT2s*abs(w + l_m*p + q_0*q_1*v_y_wind*2.0 - q_0*q_2*v_x_wind*2.0 - q_1*q_3*v_x_wind*2.0 - q_2*q_3*v_y_wind*2.0)*(q_0*q_2*2.0 + q_1*q_3*2.0) + CT2s*abs(w + l_m*q + q_0*q_1*v_y_wind*2.0 - q_0*q_2*v_x_wind*2.0 - q_1*q_3*v_x_wind*2.0 - q_2*q_3*v_y_wind*2.0)*(q_0*q_2*2.0 + q_1*q_3*2.0) + CT1s*w_1*(q_0*q_2*2.0 + q_1*q_3*2.0) + CT1s*w_2*(q_0*q_2*2.0 + q_1*q_3*2.0) + CT1s*w_3*(q_0*q_2*2.0 + q_1*q_3*2.0) + CT1s*w_4*(q_0*q_2*2.0 + q_1*q_3*2.0) + CT2s*((( - w + l_m*p - q_0*q_1*v_y_wind*2.0 + q_0*q_2*v_x_wind*2.0 + q_1*q_3*v_x_wind*2.0 + q_2*q_3*v_y_wind*2.0)/abs( - w + l_m*p - q_0*q_1*v_y_wind*2.0 + q_0*q_2*v_x_wind*2.0 + q_1*q_3*v_x_wind*2.0 + q_2*q_3*v_y_wind*2.0)))*(q_0*q_2*2.0 + q_1*q_3*2.0)*( - w + l_m*p - q_0*q_1*v_y_wind*2.0 + q_0*q_2*v_x_wind*2.0 + q_1*q_3*v_x_wind*2.0 + q_2*q_3*v_y_wind*2.0) + CT2s*((( - w + l_m*q - q_0*q_1*v_y_wind*2.0 + q_0*q_2*v_x_wind*2.0 + q_1*q_3*v_x_wind*2.0 + q_2*q_3*v_y_wind*2.0)/abs( - w + l_m*q - q_0*q_1*v_y_wind*2.0 + q_0*q_2*v_x_wind*2.0 + q_1*q_3*v_x_wind*2.0 + q_2*q_3*v_y_wind*2.0)))*(q_0*q_2*2.0 + q_1*q_3*2.0)*( - w + l_m*q - q_0*q_1*v_y_wind*2.0 + q_0*q_2*v_x_wind*2.0 + q_1*q_3*v_x_wind*2.0 + q_2*q_3*v_y_wind*2.0) + CT2s*(((w + l_m*p + q_0*q_1*v_y_wind*2.0 - q_0*q_2*v_x_wind*2.0 - q_1*q_3*v_x_wind*2.0 - q_2*q_3*v_y_wind*2.0)/abs(w + l_m*p + q_0*q_1*v_y_wind*2.0 - q_0*q_2*v_x_wind*2.0 - q_1*q_3*v_x_wind*2.0 - q_2*q_3*v_y_wind*2.0)))*(q_0*q_2*2.0 + q_1*q_3*2.0)*(w + l_m*p + q_0*q_1*v_y_wind*2.0 - q_0*q_2*v_x_wind*2.0 - q_1*q_3*v_x_wind*2.0 - q_2*q_3*v_y_wind*2.0) + CT2s*(((w + l_m*q + q_0*q_1*v_y_wind*2.0 - q_0*q_2*v_x_wind*2.0 - q_1*q_3*v_x_wind*2.0 - q_2*q_3*v_y_wind*2.0)/abs(w + l_m*q + q_0*q_1*v_y_wind*2.0 - q_0*q_2*v_x_wind*2.0 - q_1*q_3*v_x_wind*2.0 - q_2*q_3*v_y_wind*2.0)))*(q_0*q_2*2.0 + q_1*q_3*2.0)*(w + l_m*q + q_0*q_1*v_y_wind*2.0 - q_0*q_2*v_x_wind*2.0 - q_1*q_3*v_x_wind*2.0 - q_2*q_3*v_y_wind*2.0))/m + (C_wz*(q_0*q_2*2.0 + q_1*q_3*2.0)*velocityLength)/m - (C_wz*(vz_res)*1.0/velocityLength*((q_0*q_3*2.0 - q_1*q_2*2.0)*(vy_res)*2.0 - (q_0*q_2*2.0 + q_1*q_3*2.0)*(vz_res)*2.0 + (vx_res)*(q_0*q_0 + q_1*q_1 - q_2*q_2 - q_3*q_3)*2.0)*(1.0/2.0))/m;
    %     C(3,30) = (CT2s*abs( - w + l_m*p - q_0*q_1*v_y_wind*2.0 + q_0*q_2*v_x_wind*2.0 + q_1*q_3*v_x_wind*2.0 + q_2*q_3*v_y_wind*2.0)*(q_0*q_1*2.0 - q_2*q_3*2.0) + CT2s*abs( - w + l_m*q - q_0*q_1*v_y_wind*2.0 + q_0*q_2*v_x_wind*2.0 + q_1*q_3*v_x_wind*2.0 + q_2*q_3*v_y_wind*2.0)*(q_0*q_1*2.0 - q_2*q_3*2.0) + CT2s*abs(w + l_m*p + q_0*q_1*v_y_wind*2.0 - q_0*q_2*v_x_wind*2.0 - q_1*q_3*v_x_wind*2.0 - q_2*q_3*v_y_wind*2.0)*(q_0*q_1*2.0 - q_2*q_3*2.0) + CT2s*abs(w + l_m*q + q_0*q_1*v_y_wind*2.0 - q_0*q_2*v_x_wind*2.0 - q_1*q_3*v_x_wind*2.0 - q_2*q_3*v_y_wind*2.0)*(q_0*q_1*2.0 - q_2*q_3*2.0) + CT1s*w_1*(q_0*q_1*2.0 - q_2*q_3*2.0) + CT1s*w_2*(q_0*q_1*2.0 - q_2*q_3*2.0) + CT1s*w_3*(q_0*q_1*2.0 - q_2*q_3*2.0) + CT1s*w_4*(q_0*q_1*2.0 - q_2*q_3*2.0) + CT2s*((( - w + l_m*p - q_0*q_1*v_y_wind*2.0 + q_0*q_2*v_x_wind*2.0 + q_1*q_3*v_x_wind*2.0 + q_2*q_3*v_y_wind*2.0)/abs( - w + l_m*p - q_0*q_1*v_y_wind*2.0 + q_0*q_2*v_x_wind*2.0 + q_1*q_3*v_x_wind*2.0 + q_2*q_3*v_y_wind*2.0)))*(q_0*q_1*2.0 - q_2*q_3*2.0)*( - w + l_m*p - q_0*q_1*v_y_wind*2.0 + q_0*q_2*v_x_wind*2.0 + q_1*q_3*v_x_wind*2.0 + q_2*q_3*v_y_wind*2.0) + CT2s*((( - w + l_m*q - q_0*q_1*v_y_wind*2.0 + q_0*q_2*v_x_wind*2.0 + q_1*q_3*v_x_wind*2.0 + q_2*q_3*v_y_wind*2.0)/abs( - w + l_m*q - q_0*q_1*v_y_wind*2.0 + q_0*q_2*v_x_wind*2.0 + q_1*q_3*v_x_wind*2.0 + q_2*q_3*v_y_wind*2.0)))*(q_0*q_1*2.0 - q_2*q_3*2.0)*( - w + l_m*q - q_0*q_1*v_y_wind*2.0 + q_0*q_2*v_x_wind*2.0 + q_1*q_3*v_x_wind*2.0 + q_2*q_3*v_y_wind*2.0) + CT2s*(((w + l_m*p + q_0*q_1*v_y_wind*2.0 - q_0*q_2*v_x_wind*2.0 - q_1*q_3*v_x_wind*2.0 - q_2*q_3*v_y_wind*2.0)/abs(w + l_m*p + q_0*q_1*v_y_wind*2.0 - q_0*q_2*v_x_wind*2.0 - q_1*q_3*v_x_wind*2.0 - q_2*q_3*v_y_wind*2.0)))*(q_0*q_1*2.0 - q_2*q_3*2.0)*(w + l_m*p + q_0*q_1*v_y_wind*2.0 - q_0*q_2*v_x_wind*2.0 - q_1*q_3*v_x_wind*2.0 - q_2*q_3*v_y_wind*2.0) + CT2s*(((w + l_m*q + q_0*q_1*v_y_wind*2.0 - q_0*q_2*v_x_wind*2.0 - q_1*q_3*v_x_wind*2.0 - q_2*q_3*v_y_wind*2.0)/abs(w + l_m*q + q_0*q_1*v_y_wind*2.0 - q_0*q_2*v_x_wind*2.0 - q_1*q_3*v_x_wind*2.0 - q_2*q_3*v_y_wind*2.0)))*(q_0*q_1*2.0 - q_2*q_3*2.0)*(w + l_m*q + q_0*q_1*v_y_wind*2.0 - q_0*q_2*v_x_wind*2.0 - q_1*q_3*v_x_wind*2.0 - q_2*q_3*v_y_wind*2.0))/m - (C_wz*(q_0*q_1*2.0 - q_2*q_3*2.0)*velocityLength)/m - (C_wz*(vz_res)*1.0/velocityLength*((q_0*q_3*2.0 + q_1*q_2*2.0)*(vx_res)*2.0 - (vy_res)*(q_0*q_0 - q_1*q_1 + q_2*q_2 - q_3*q_3)*2.0 + (q_0*q_1*2.0 - q_2*q_3*2.0)*(vz_res)*2.0)*(1.0/2.0))/m;
end
% C(1,18) =  - w;
% C(1,19) = v;
% C(1,29) = (C_wxy*velocityLength*(q_0*q_0 + q_1*q_1 - q_2*q_2 - q_3*q_3))/m + (C_wxy*(vx_res)*1.0/velocityLength*((q_0*q_3*2.0 - q_1*q_2*2.0)*(vy_res)*2.0 - (q_0*q_2*2.0 + q_1*q_3*2.0)*(vz_res)*2.0 + (vx_res)*(q_0*q_0 + q_1*q_1 - q_2*q_2 - q_3*q_3)*2.0)*(1.0/2.0))/m;
% C(1,30) = (C_wxy*(q_0*q_3*2.0 + q_1*q_2*2.0)*velocityLength)/m + (C_wxy*(vx_res)*1.0/velocityLength*((q_0*q_3*2.0 + q_1*q_2*2.0)*(vx_res)*2.0 - (vy_res)*(q_0*q_0 - q_1*q_1 + q_2*q_2 - q_3*q_3)*2.0 + (q_0*q_1*2.0 - q_2*q_3*2.0)*(vz_res)*2.0)*(1.0/2.0))/m;
% C(1,31) = ((vx_res)*velocityLength)/m;
% C(2,17) = w;
% C(2,19) =  - u;
% C(2,29) =  - (C_wxy*(q_0*q_3*2.0 - q_1*q_2*2.0)*velocityLength)/m - (C_wxy*1.0/velocityLength*(vy_res)*((q_0*q_3*2.0 - q_1*q_2*2.0)*(vy_res)*2.0 - (q_0*q_2*2.0 + q_1*q_3*2.0)*(vz_res)*2.0 + (vx_res)*(q_0*q_0 + q_1*q_1 - q_2*q_2 - q_3*q_3)*2.0)*(1.0/2.0))/m;
% C(2,30) = (C_wxy*velocityLength*(q_0*q_0 - q_1*q_1 + q_2*q_2 - q_3*q_3))/m - (C_wxy*1.0/velocityLength*(vy_res)*((q_0*q_3*2.0 + q_1*q_2*2.0)*(vx_res)*2.0 - (vy_res)*(q_0*q_0 - q_1*q_1 + q_2*q_2 - q_3*q_3)*2.0 + (q_0*q_1*2.0 - q_2*q_3*2.0)*(vz_res)*2.0)*(1.0/2.0))/m;
% C(2,31) =  - (velocityLength*(vy_res))/m;
% C(3,17) =  - v + (CT2s*l_m*abs(w + l_m*p + q_0*q_1*v_y_wind*2.0 - q_0*q_2*v_x_wind*2.0 - q_1*q_3*v_x_wind*2.0 - q_2*q_3*v_y_wind*2.0) + CT1s*l_m*w_2 - CT1s*l_m*w_4 - CT2s*l_m*abs( - w + l_m*p - q_0*q_1*v_y_wind*2.0 + q_0*q_2*v_x_wind*2.0 + q_1*q_3*v_x_wind*2.0 + q_2*q_3*v_y_wind*2.0) - CT2s*l_m*((( - w + l_m*p - q_0*q_1*v_y_wind*2.0 + q_0*q_2*v_x_wind*2.0 + q_1*q_3*v_x_wind*2.0 + q_2*q_3*v_y_wind*2.0)/abs( - w + l_m*p - q_0*q_1*v_y_wind*2.0 + q_0*q_2*v_x_wind*2.0 + q_1*q_3*v_x_wind*2.0 + q_2*q_3*v_y_wind*2.0)))*( - w + l_m*p - q_0*q_1*v_y_wind*2.0 + q_0*q_2*v_x_wind*2.0 + q_1*q_3*v_x_wind*2.0 + q_2*q_3*v_y_wind*2.0) + CT2s*l_m*(((w + l_m*p + q_0*q_1*v_y_wind*2.0 - q_0*q_2*v_x_wind*2.0 - q_1*q_3*v_x_wind*2.0 - q_2*q_3*v_y_wind*2.0)/abs(w + l_m*p + q_0*q_1*v_y_wind*2.0 - q_0*q_2*v_x_wind*2.0 - q_1*q_3*v_x_wind*2.0 - q_2*q_3*v_y_wind*2.0)))*(w + l_m*p + q_0*q_1*v_y_wind*2.0 - q_0*q_2*v_x_wind*2.0 - q_1*q_3*v_x_wind*2.0 - q_2*q_3*v_y_wind*2.0))/m;
% C(3,18) = u + (CT2s*l_m*abs(w + l_m*q + q_0*q_1*v_y_wind*2.0 - q_0*q_2*v_x_wind*2.0 - q_1*q_3*v_x_wind*2.0 - q_2*q_3*v_y_wind*2.0) - CT1s*l_m*w_1 + CT1s*l_m*w_3 - CT2s*l_m*abs( - w + l_m*q - q_0*q_1*v_y_wind*2.0 + q_0*q_2*v_x_wind*2.0 + q_1*q_3*v_x_wind*2.0 + q_2*q_3*v_y_wind*2.0) - CT2s*l_m*((( - w + l_m*q - q_0*q_1*v_y_wind*2.0 + q_0*q_2*v_x_wind*2.0 + q_1*q_3*v_x_wind*2.0 + q_2*q_3*v_y_wind*2.0)/abs( - w + l_m*q - q_0*q_1*v_y_wind*2.0 + q_0*q_2*v_x_wind*2.0 + q_1*q_3*v_x_wind*2.0 + q_2*q_3*v_y_wind*2.0)))*( - w + l_m*q - q_0*q_1*v_y_wind*2.0 + q_0*q_2*v_x_wind*2.0 + q_1*q_3*v_x_wind*2.0 + q_2*q_3*v_y_wind*2.0) + CT2s*l_m*(((w + l_m*q + q_0*q_1*v_y_wind*2.0 - q_0*q_2*v_x_wind*2.0 - q_1*q_3*v_x_wind*2.0 - q_2*q_3*v_y_wind*2.0)/abs(w + l_m*q + q_0*q_1*v_y_wind*2.0 - q_0*q_2*v_x_wind*2.0 - q_1*q_3*v_x_wind*2.0 - q_2*q_3*v_y_wind*2.0)))*(w + l_m*q + q_0*q_1*v_y_wind*2.0 - q_0*q_2*v_x_wind*2.0 - q_1*q_3*v_x_wind*2.0 - q_2*q_3*v_y_wind*2.0))/m;
% C(3,20) =  - (CT0s*w_1*2.0 + CT1s*( - w + l_m*q - q_0*q_1*v_y_wind*2.0 + q_0*q_2*v_x_wind*2.0 + q_1*q_3*v_x_wind*2.0 + q_2*q_3*v_y_wind*2.0))/m;
% C(3,21) =  - (CT0s*w_2*2.0 - CT1s*(w + l_m*p + q_0*q_1*v_y_wind*2.0 - q_0*q_2*v_x_wind*2.0 - q_1*q_3*v_x_wind*2.0 - q_2*q_3*v_y_wind*2.0))/m;
% C(3,22) =  - (CT0s*w_3*2.0 - CT1s*(w + l_m*q + q_0*q_1*v_y_wind*2.0 - q_0*q_2*v_x_wind*2.0 - q_1*q_3*v_x_wind*2.0 - q_2*q_3*v_y_wind*2.0))/m;
% C(3,23) =  - (CT0s*w_4*2.0 + CT1s*( - w + l_m*p - q_0*q_1*v_y_wind*2.0 + q_0*q_2*v_x_wind*2.0 + q_1*q_3*v_x_wind*2.0 + q_2*q_3*v_y_wind*2.0))/m;
% C(3,25) =  - (w_1*w_1 + w_2*w_2 + w_3*w_3 + w_4*w_4)/m;
% C(3,29) =  - (CT2s*abs( - w + l_m*p - q_0*q_1*v_y_wind*2.0 + q_0*q_2*v_x_wind*2.0 + q_1*q_3*v_x_wind*2.0 + q_2*q_3*v_y_wind*2.0)*(q_0*q_2*2.0 + q_1*q_3*2.0) + CT2s*abs( - w + l_m*q - q_0*q_1*v_y_wind*2.0 + q_0*q_2*v_x_wind*2.0 + q_1*q_3*v_x_wind*2.0 + q_2*q_3*v_y_wind*2.0)*(q_0*q_2*2.0 + q_1*q_3*2.0) + CT2s*abs(w + l_m*p + q_0*q_1*v_y_wind*2.0 - q_0*q_2*v_x_wind*2.0 - q_1*q_3*v_x_wind*2.0 - q_2*q_3*v_y_wind*2.0)*(q_0*q_2*2.0 + q_1*q_3*2.0) + CT2s*abs(w + l_m*q + q_0*q_1*v_y_wind*2.0 - q_0*q_2*v_x_wind*2.0 - q_1*q_3*v_x_wind*2.0 - q_2*q_3*v_y_wind*2.0)*(q_0*q_2*2.0 + q_1*q_3*2.0) + CT1s*w_1*(q_0*q_2*2.0 + q_1*q_3*2.0) + CT1s*w_2*(q_0*q_2*2.0 + q_1*q_3*2.0) + CT1s*w_3*(q_0*q_2*2.0 + q_1*q_3*2.0) + CT1s*w_4*(q_0*q_2*2.0 + q_1*q_3*2.0) + CT2s*((( - w + l_m*p - q_0*q_1*v_y_wind*2.0 + q_0*q_2*v_x_wind*2.0 + q_1*q_3*v_x_wind*2.0 + q_2*q_3*v_y_wind*2.0)/abs( - w + l_m*p - q_0*q_1*v_y_wind*2.0 + q_0*q_2*v_x_wind*2.0 + q_1*q_3*v_x_wind*2.0 + q_2*q_3*v_y_wind*2.0)))*(q_0*q_2*2.0 + q_1*q_3*2.0)*( - w + l_m*p - q_0*q_1*v_y_wind*2.0 + q_0*q_2*v_x_wind*2.0 + q_1*q_3*v_x_wind*2.0 + q_2*q_3*v_y_wind*2.0) + CT2s*((( - w + l_m*q - q_0*q_1*v_y_wind*2.0 + q_0*q_2*v_x_wind*2.0 + q_1*q_3*v_x_wind*2.0 + q_2*q_3*v_y_wind*2.0)/abs( - w + l_m*q - q_0*q_1*v_y_wind*2.0 + q_0*q_2*v_x_wind*2.0 + q_1*q_3*v_x_wind*2.0 + q_2*q_3*v_y_wind*2.0)))*(q_0*q_2*2.0 + q_1*q_3*2.0)*( - w + l_m*q - q_0*q_1*v_y_wind*2.0 + q_0*q_2*v_x_wind*2.0 + q_1*q_3*v_x_wind*2.0 + q_2*q_3*v_y_wind*2.0) + CT2s*(((w + l_m*p + q_0*q_1*v_y_wind*2.0 - q_0*q_2*v_x_wind*2.0 - q_1*q_3*v_x_wind*2.0 - q_2*q_3*v_y_wind*2.0)/abs(w + l_m*p + q_0*q_1*v_y_wind*2.0 - q_0*q_2*v_x_wind*2.0 - q_1*q_3*v_x_wind*2.0 - q_2*q_3*v_y_wind*2.0)))*(q_0*q_2*2.0 + q_1*q_3*2.0)*(w + l_m*p + q_0*q_1*v_y_wind*2.0 - q_0*q_2*v_x_wind*2.0 - q_1*q_3*v_x_wind*2.0 - q_2*q_3*v_y_wind*2.0) + CT2s*(((w + l_m*q + q_0*q_1*v_y_wind*2.0 - q_0*q_2*v_x_wind*2.0 - q_1*q_3*v_x_wind*2.0 - q_2*q_3*v_y_wind*2.0)/abs(w + l_m*q + q_0*q_1*v_y_wind*2.0 - q_0*q_2*v_x_wind*2.0 - q_1*q_3*v_x_wind*2.0 - q_2*q_3*v_y_wind*2.0)))*(q_0*q_2*2.0 + q_1*q_3*2.0)*(w + l_m*q + q_0*q_1*v_y_wind*2.0 - q_0*q_2*v_x_wind*2.0 - q_1*q_3*v_x_wind*2.0 - q_2*q_3*v_y_wind*2.0))/m + (C_wz*(q_0*q_2*2.0 + q_1*q_3*2.0)*velocityLength)/m - (C_wz*(vz_res)*1.0/velocityLength*((q_0*q_3*2.0 - q_1*q_2*2.0)*(vy_res)*2.0 - (q_0*q_2*2.0 + q_1*q_3*2.0)*(vz_res)*2.0 + (vx_res)*(q_0*q_0 + q_1*q_1 - q_2*q_2 - q_3*q_3)*2.0)*(1.0/2.0))/m;
% C(3,30) = (CT2s*abs( - w + l_m*p - q_0*q_1*v_y_wind*2.0 + q_0*q_2*v_x_wind*2.0 + q_1*q_3*v_x_wind*2.0 + q_2*q_3*v_y_wind*2.0)*(q_0*q_1*2.0 - q_2*q_3*2.0) + CT2s*abs( - w + l_m*q - q_0*q_1*v_y_wind*2.0 + q_0*q_2*v_x_wind*2.0 + q_1*q_3*v_x_wind*2.0 + q_2*q_3*v_y_wind*2.0)*(q_0*q_1*2.0 - q_2*q_3*2.0) + CT2s*abs(w + l_m*p + q_0*q_1*v_y_wind*2.0 - q_0*q_2*v_x_wind*2.0 - q_1*q_3*v_x_wind*2.0 - q_2*q_3*v_y_wind*2.0)*(q_0*q_1*2.0 - q_2*q_3*2.0) + CT2s*abs(w + l_m*q + q_0*q_1*v_y_wind*2.0 - q_0*q_2*v_x_wind*2.0 - q_1*q_3*v_x_wind*2.0 - q_2*q_3*v_y_wind*2.0)*(q_0*q_1*2.0 - q_2*q_3*2.0) + CT1s*w_1*(q_0*q_1*2.0 - q_2*q_3*2.0) + CT1s*w_2*(q_0*q_1*2.0 - q_2*q_3*2.0) + CT1s*w_3*(q_0*q_1*2.0 - q_2*q_3*2.0) + CT1s*w_4*(q_0*q_1*2.0 - q_2*q_3*2.0) + CT2s*((( - w + l_m*p - q_0*q_1*v_y_wind*2.0 + q_0*q_2*v_x_wind*2.0 + q_1*q_3*v_x_wind*2.0 + q_2*q_3*v_y_wind*2.0)/abs( - w + l_m*p - q_0*q_1*v_y_wind*2.0 + q_0*q_2*v_x_wind*2.0 + q_1*q_3*v_x_wind*2.0 + q_2*q_3*v_y_wind*2.0)))*(q_0*q_1*2.0 - q_2*q_3*2.0)*( - w + l_m*p - q_0*q_1*v_y_wind*2.0 + q_0*q_2*v_x_wind*2.0 + q_1*q_3*v_x_wind*2.0 + q_2*q_3*v_y_wind*2.0) + CT2s*((( - w + l_m*q - q_0*q_1*v_y_wind*2.0 + q_0*q_2*v_x_wind*2.0 + q_1*q_3*v_x_wind*2.0 + q_2*q_3*v_y_wind*2.0)/abs( - w + l_m*q - q_0*q_1*v_y_wind*2.0 + q_0*q_2*v_x_wind*2.0 + q_1*q_3*v_x_wind*2.0 + q_2*q_3*v_y_wind*2.0)))*(q_0*q_1*2.0 - q_2*q_3*2.0)*( - w + l_m*q - q_0*q_1*v_y_wind*2.0 + q_0*q_2*v_x_wind*2.0 + q_1*q_3*v_x_wind*2.0 + q_2*q_3*v_y_wind*2.0) + CT2s*(((w + l_m*p + q_0*q_1*v_y_wind*2.0 - q_0*q_2*v_x_wind*2.0 - q_1*q_3*v_x_wind*2.0 - q_2*q_3*v_y_wind*2.0)/abs(w + l_m*p + q_0*q_1*v_y_wind*2.0 - q_0*q_2*v_x_wind*2.0 - q_1*q_3*v_x_wind*2.0 - q_2*q_3*v_y_wind*2.0)))*(q_0*q_1*2.0 - q_2*q_3*2.0)*(w + l_m*p + q_0*q_1*v_y_wind*2.0 - q_0*q_2*v_x_wind*2.0 - q_1*q_3*v_x_wind*2.0 - q_2*q_3*v_y_wind*2.0) + CT2s*(((w + l_m*q + q_0*q_1*v_y_wind*2.0 - q_0*q_2*v_x_wind*2.0 - q_1*q_3*v_x_wind*2.0 - q_2*q_3*v_y_wind*2.0)/abs(w + l_m*q + q_0*q_1*v_y_wind*2.0 - q_0*q_2*v_x_wind*2.0 - q_1*q_3*v_x_wind*2.0 - q_2*q_3*v_y_wind*2.0)))*(q_0*q_1*2.0 - q_2*q_3*2.0)*(w + l_m*q + q_0*q_1*v_y_wind*2.0 - q_0*q_2*v_x_wind*2.0 - q_1*q_3*v_x_wind*2.0 - q_2*q_3*v_y_wind*2.0))/m - (C_wz*(q_0*q_1*2.0 - q_2*q_3*2.0)*velocityLength)/m - (C_wz*(vz_res)*1.0/velocityLength*((q_0*q_3*2.0 + q_1*q_2*2.0)*(vx_res)*2.0 - (vy_res)*(q_0*q_0 - q_1*q_1 + q_2*q_2 - q_3*q_3)*2.0 + (q_0*q_1*2.0 - q_2*q_3*2.0)*(vz_res)*2.0)*(1.0/2.0))/m;

R        = diag(Rin);

temp = real_measurements  -  y;

function [temp,C,R] = getGyroscope(x,real_measurements,Rin)

%% Initial conditions
p_bias = x(14);
q_bias = x(15);
r_bias = x(16);
p = x(17);
q = x(18);
r = x(19);

y   = zeros(3,1);
C   = zeros(3,31);

y(1) = p + p_bias;
y(2) = q + q_bias;
y(3) = r + r_bias;

C(1,14) = 1.0;
C(1,17) = 1.0;
C(2,15) = 1.0;
C(2,18) = 1.0;
C(3,16) = 1.0;
C(3,19) = 1.0;

R       = diag(Rin);

temp = real_measurements  -  y;

function [temp,C,R] = getOmegaMotor(x,real_measurements,Rin)

%% Initial conditions

w_1 = x(20);
w_2 = x(21);
w_3 = x(22);
w_4 = x(23);

y    = zeros(4,1);
C    = zeros(4,31);

y(1) = w_1;
y(2) = w_2;
y(3) = w_3;
y(4) = w_4;

C(1,20) = 1.0;
C(2,21) = 1.0;
C(3,22) = 1.0;
C(4,23) = 1.0;

R       = diag(Rin);

temp = real_measurements  -  y;
